simulink model "batt"  (R2021a)
settings: Solver=VariableStepAuto  StartTime=0.0  StopTime=0.2  RelTol=1e-3
undefined symbols (not defined in the file): Acid, Lead
libraries: spsIGBTDiodeLib x6, spsSeriesRLCBranchLib x3, spsVoltageMeasurementLib x3, spsCurrentMeasurementLib x2, spsBatteryLib x1, spsACVoltageSourceLib x1, pid_lib x1, spsPLLLib x1, spsPWMGeneratorDCDCLib x1, spspowerguiLib x1
settings Model: Creator=User  LastModifiedBy=User

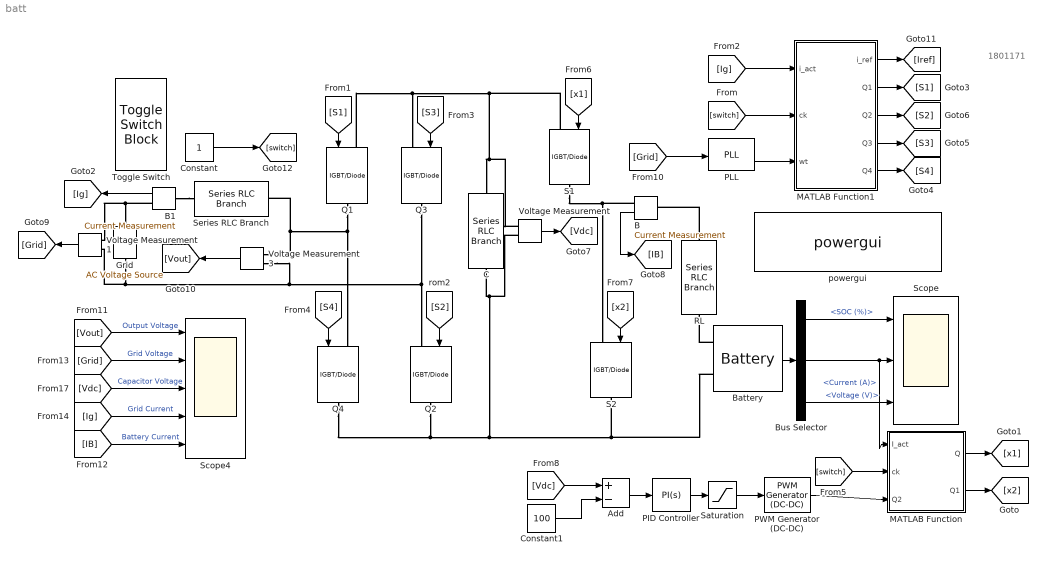
== system batt ==
  note: 1801171
  Add : Sum  Inputs=+-
  B : spsCurrentMeasurementLib/Current Measurement  PhasorSimulation=off  OutputType=Complex  PSBequivalent=0
  B1 : spsCurrentMeasurementLib/Current Measurement  PhasorSimulation=off  OutputType=Complex  PSBequivalent=0
  Battery : spsBatteryLib/Battery  BatType=Lead-Acid  ShowTempParam=off  ThermalPreset=no  ShowAgeParam=off  NomV=60  NomQ=10  SOC=70  Batt_Tr=30  PresetModel=on  MaxQ=10.4167  MinV=45  FullV=65.3289  Dis_rate=2  R=0.06  Normal_OP=3.1028  expZone="[61.0855    0.0333333]"  current=[6.5 13 32.5]  Units=Time  Tci=20  NomT=20  T2=-30  MaxQ2=4.8  FullV2=7.1  Normal_OP2=5.655  expZone2="[6.58           1]"  Rca=0.6  ti=2000  Dp=0  Neq0=0  Tsim=1e6  Ta1=25  Qeol=5.4*0.9  Reol=0.013333*1.2  Char_age=[2.3478, 3]  Dis_age=[2.3478, 10]  N1=1500  N2=10500  N3=1000  N4=1400  Ta2=45  N5=950
  Bus Selector : BusSelector  OutputSignals=SOC (%),Current (A),Voltage (V)
  C : spsSeriesRLCBranchLib/Series RLC Branch  LConnTagsString=__new0  RConnTagsString=__new0  BranchType=C  Resistance=.1  Inductance=5e-3  SetiL0=off  InitialCurrent=0  Capacitance=1000e-6  Setx0=off  InitialVoltage=0  Measurements=None
  Constant : Constant
  Constant1 : Constant  Value=100
  Grid : spsACVoltageSourceLib/AC Voltage Source  Amplitude=100  Phase=0  Frequency=50  SampleTime=0  Measurements=None  BusType=swing  Pref=10e3  Qref=0  Qmin=-inf  Qmax=+inf
  MATLAB Function : MATLAB Function  TreatAsAtomicUnit=on
  MATLAB Function1 : MATLAB Function  TreatAsAtomicUnit=on
  PID Controller : pid_lib/PID Controller  Controller=PI  Form=Parallel  TimeDomain=Continuous-time  UseExternalTs=off  SampleTime=-1  IntegratorMethod=Forward Euler  FilterMethod=Forward Euler  ControllerParametersSource=internal  P=0.1  I=0.01  D=0  UseFilter=on  N=100  TunerSelectOption=Transfer Function Based (PID Tuner App)  InitialConditionSource=internal  InitialConditionForIntegrator=0  InitialConditionForFilter=0  DifferentiatorICPrevScaledInput=0  ExternalReset=none  TrackingMode=off  Kt=1  LimitOutput=off  SatLimitsSource=internal  UpperSaturationLimit=inf  LowerSaturationLimit=-inf  LinearizeAsGain=on  AntiWindupMode=none  Kb=1  POutMin=[]  POutMax=[]  IOutMin=[]  IOutMax=[]  DOutMin=[]  DOutMax=[]  NOutMin=[]  NOutMax=[]  SumOutMin=[]  SumOutMax=[]  SaturationOutMin=[]  SaturationOutMax=[]  PParamMin=[]  PParamMax=[]  IParamMin=[]  IParamMax=[]  DParamMin=[]  DParamMax=[]  NParamMin=[]  NParamMax=[]  KbParamMin=[]  KbParamMax=[]  KtParamMin=[]  KtParamMax=[]  KbOutMin=[]  KbOutMax=[]  KtOutMin=[]  KtOutMax=[]  IntegratorOutMin=[]  IntegratorOutMax=[]  FilterOutMin=[]  FilterOutMax=[]  SumI1OutMin=[]  SumI1OutMax=[]  SumI2OutMin=[]  SumI2OutMax=[]  SumI3OutMin=[]  SumI3OutMax=[]  SumI4OutMin=[]  SumI4OutMax=[]  SumDOutMin=[]  SumDOutMax=[]  DifferentiatorOutMin=[]  DifferentiatorOutMax=[]  FilterDiffOutCoefMin=[]  FilterDiffOutCoefMax=[]  ReciprocalOutMin=[]  ReciprocalOutMax=[]  SumDenOutMin=[]  SumDenOutMax=[]  SumNumOutMin=[]  SumNumOutMax=[]  DivideOutMin=[]  DivideOutMax=[]  UdiffTsProdOutMin=[]  UdiffTsProdOutMax=[]  NTsProdOutMin=[]  NTsProdOutMax=[]  UintegralTsProdOutMin=[]  UintegralTsProdOutMax=[]  UngainTsProdOutMin=[]  UngainTsProdOutMax=[]  IntegratorContinuousStateAttributes=''  IntegratorStateMustResolveToSignalObject=off  IntegratorRTWStateStorageClass=Auto  FilterContinuousStateAttributes=''  FilterStateMustResolveToSignalObject=off  FilterRTWStateStorageClass=Auto  ParallelPVariant=InternalParameters  IdealPVariant=Disabled  IVariant=InternalParameters  DVariant=Disabled  IntegratorVariant=Continuous  SatVariant=Disabled  AWVariant=Passthrough  PCopyVariant=Disabled  TRVariant=Disabled  FdbkBlocksVariant=Forward  IdealPFdbkVariant=Disabled  SatFdbkVariant=Disabled  DerivativeFilterVariant=Disabled  NVariant=Disabled  NCopyVariant=Disabled_SignalSpec  FilterICVariant=Disabled  IntegratorICVariant=InternalICs  ExternalResetVariant=Disabled  TRSumVariant=Passthrough  SumFdbkVariant=Disabled  SumVariant=Sum_PI  TsampFilterVariant=InternalTs  TsampNgainVariant=Passthrough  TsampIntegralVariant=Passthrough  ExternalSaturationOutDataTypeStr=Inherit: Same as second input
  PLL : spsPLLLib/PLL  Fmin=45  Par_Init=[0, 50]  ParK=[180, 3200, 1]  TcD=1e-4  MaxRateChangeFreq=12  FilterCutOffFreq=25  Ts=0  AGC=on
      settings: SourceProductBaseCode=PS
  PWM Generator (DC-DC) : spsPWMGeneratorDCDCLib/PWM Generator (DC-DC)  Fsw=5000  Ts=0
  Q{1..4} (4 alike) : spsIGBTDiodeLib/IGBT//Diode  Ron=1e-3  Rs=1e5  Cs=inf  Measurements=off
  RL : spsSeriesRLCBranchLib/Series RLC Branch  LConnTagsString=__new0  RConnTagsString=__new0  BranchType=RL  Resistance=.1  Inductance=5e-3  SetiL0=off  InitialCurrent=0  Capacitance=1e-6  Setx0=off  InitialVoltage=0  Measurements=None
  S1 : spsIGBTDiodeLib/IGBT//Diode  Ron=1e-3  Rs=1e5  Cs=inf  Measurements=off
  S2 : spsIGBTDiodeLib/IGBT//Diode  Ron=1e-3  Rs=1e5  Cs=inf  Measurements=off
  Saturation : Saturate  LowerLimit=0
  Scope : Scope  NumInputPorts=3
  Scope4 : Scope  NumInputPorts=5
  Series RLC Branch : spsSeriesRLCBranchLib/Series RLC Branch  LConnTagsString=__new0  RConnTagsString=__new0  BranchType=RL  Resistance=.1  Inductance=5e-3  SetiL0=off  InitialCurrent=0  Capacitance=1e-6  Setx0=off  InitialVoltage=0  Measurements=None
  Toggle Switch : ToggleSwitchBlock
      settings: Values={{'Off', 'On'}, [0 1]}
  Voltage Measurement : spsVoltageMeasurementLib/Voltage Measurement  PhasorSimulation=off  OutputType=Complex  PSBequivalent=0
  Voltage Measurement1 : spsVoltageMeasurementLib/Voltage Measurement  PhasorSimulation=off  OutputType=Complex  PSBequivalent=0
  Voltage Measurement3 : spsVoltageMeasurementLib/Voltage Measurement  PhasorSimulation=off  OutputType=Complex  PSBequivalent=0
  powergui : spspowerguiLib/powergui  Priority=1  SimulationMode=Discrete  SampleTime=50e-6  frequency=60  Iterations=50  frequencyindice=0  Pbase=100e6  ErrMax=1e-4  UnitsV=kV  UnitsW=MW  buscounter=0  FunctionMessages=off  echomessages=off  EnableUseOfTLC=off  CurrentSourceSwitches=off  DisableSnubberDevices=off  DisableRonSwitches=off  DisableVfSwitches=off  DisplayEquations=off  AutomaticDiscreteSolvers=off  SolverType=Tustin/Backward Euler (TBE)  Interpol=off  ExternalGateDelay=off  methode=off  Ts=100  x0status=blocks  SPID=on  SwTol=0  HookPort=off  NonlinearTolerance=1e-4  nMaxIteration=100  ContinueOnMaxIteration=off  RestoreLinks=warning  ResistiveCurrentMeasurement=off  Frange=[0:2:500]  Ylog=off  Xlog=on  ShowGrid=off  save=off  variable=ZData  structure=0  ZoomFFT=off  StartTime=0.0  cycles=1  DisplayStyle=1  fundamental=60  FreqAxis=off  MaxFrequency=1000  frequencyindicesteady=1  RmsSteady=1  display=off
  wires:
  Bus Selector/1 -> Scope/1  "<SOC (%)>"
  Add/1 -> PID Controller/1
  PID Controller/1 -> Saturation/1
  Constant1/1 -> Add/2
  PWM Generator (DC-DC)/1 -> MATLAB Function/3(Q2)
  Saturation/1 -> PWM Generator (DC-DC)/1
  MATLAB Function1/2(Q1) -> [S1]
  [Ig] -> Scope4/4  "Grid Current"
  [Vdc] -> Add/1
  Voltage Measurement1/1 -> [Grid]
  Bus Selector/2 -> MATLAB Function/1(I_act), Scope/2  "<Current (A)>"
  Bus Selector/3 -> Scope/3  "<Voltage (V)>"
  PLL/2 -> MATLAB Function1/3(wt)
  [S3] -> Q3/1
  [switch] -> MATLAB Function/2(ck)
  Voltage Measurement3/1 -> [Vout]
  Constant/1 -> [switch]
  Voltage Measurement/1 -> [Vdc]
  [S1] -> Q1/1
  [x1] -> S1/1
  [Ig] -> MATLAB Function1/1(i_act)
  MATLAB Function1/4(Q3) -> [S3]
  B/1 -> [IB]
  [x2] -> S2/1
  MATLAB Function1/3(Q2) -> [S2]
  MATLAB Function/1(Q) -> [x1]
  B1/1 -> [Ig]
  [switch] -> MATLAB Function1/2(ck)
  MATLAB Function1/5(Q4) -> [S4]
  [Grid] -> PLL/1
  [S2] -> Q2/1
  MATLAB Function1/1(i_ref) -> [Iref]
  MATLAB Function/2(Q1) -> [x2]
  [Vout] -> Scope4/1  "Output Voltage"
  [S4] -> Q4/1
  Battery/1 -> Bus Selector/1
  [Grid] -> Scope4/2  "Grid Voltage"
  [IB] -> Scope4/5  "Battery Current"
  [Vdc] -> Scope4/3  "Capacitor Voltage"
  connections:
  Voltage Measurement/LConn2 -- C/RConn1 -- S2/RConn1 -- Battery/LConn2 -- Q4/RConn1 -- Q2/RConn1
  Voltage Measurement3/LConn2 -- Grid/LConn1 -- Voltage Measurement1/LConn2 -- Q3/RConn1 -- Q2/LConn1
  Q1/LConn1 -- Q3/LConn1 -- C/LConn1 -- Voltage Measurement/LConn1 -- S1/LConn1
  Voltage Measurement3/LConn1 -- Q1/RConn1 -- Q4/LConn1 -- Series RLC Branch/RConn1
  S1/RConn1 -- B/RConn1 -- S2/LConn1
  B1/RConn1 -- Voltage Measurement1/LConn1 -- Grid/RConn1
  Battery/LConn1 -- RL/RConn1
  B1/LConn1 -- Series RLC Branch/LConn1
  RL/LConn1 -- B/LConn1

== matlab function batt/MATLAB Function1 ==
  settings: updateMethod=DISCRETE
  data: i_ref output; i_act input; Q1 output; Q2 output; Q3 output; Q4 output; ck input; wt input
function [i_ref,Q1,Q2,Q3,Q4] = fcn(i_act,ck,wt) 
Vg = 100;
pf = .8;
P = 300;
phase = acos(pf);
ig_m=(P*sqrt(2))/(Vg*pf); 
i_ref = ig_m*sin(wt-phase); 

persistent s1
if isempty(s1) s1=0; end 
persistent s2 
if isempty(s2) s2=0; end 
persistent s3 
if isempty(s3) s3=0; end 
persistent s4 
if isempty(s4) s4=0; end 
d=0.1; 
e=i_act-i_ref;
if ck == 1
    s1 = 0; s2 =0; s3 = 0; s4 = 0;
else
    if i_ref>=0 
        if e<-d 
            s1=1; s2=1; s3=0; s4=0; 
        elseif e>d 
            s1=0; s2=0; s3=1; s4=1; 
        end 
    else 
        if e<-d 
            s1=1; s2=1; s3=0; s4=0; 
        elseif e>d 
            s1=0; s2=0; s3=1; s4=1; 
        end 
    end
end
Q1=s1; Q2=s2; Q3=s3; Q4=s4; 
end

== matlab function batt/MATLAB Function ==
  settings: updateMethod=DISCRETE
  data: I_act input; Q output; Q1 output; ck input; Q2 input
function [Q,Q1] = fcn(I_act,ck,Q2)
I_ref = 5;
d=0.1;
persistent s;if isempty(s) s = 1; end
if ck == 1
    if I_act <= -(I_ref+d)
        s = 0;
    elseif I_act >= - (I_ref-d)
        s = 1;
    else
        s=s;
    end
    Q = s; Q1 = 0;
   
else
    Q=0; Q1=Q2;
   end
end
